simulink model "Figure_1_5_TP_Telecom_demodulation"  (R2020a)
settings: Solver=FixedStepDiscrete  StartTime=0.0  StopTime=999  RelTol=1e-3
libraries: simulink x2, commrandsrc3 x1, commsink2 x1, commfilt2 x1, dspsigops x1, commutil2 x1
Description:
  | C'est un TP Télécom à faire.
settings Model: Creator=Mr Ibrahima BA  LastModifiedBy=iba

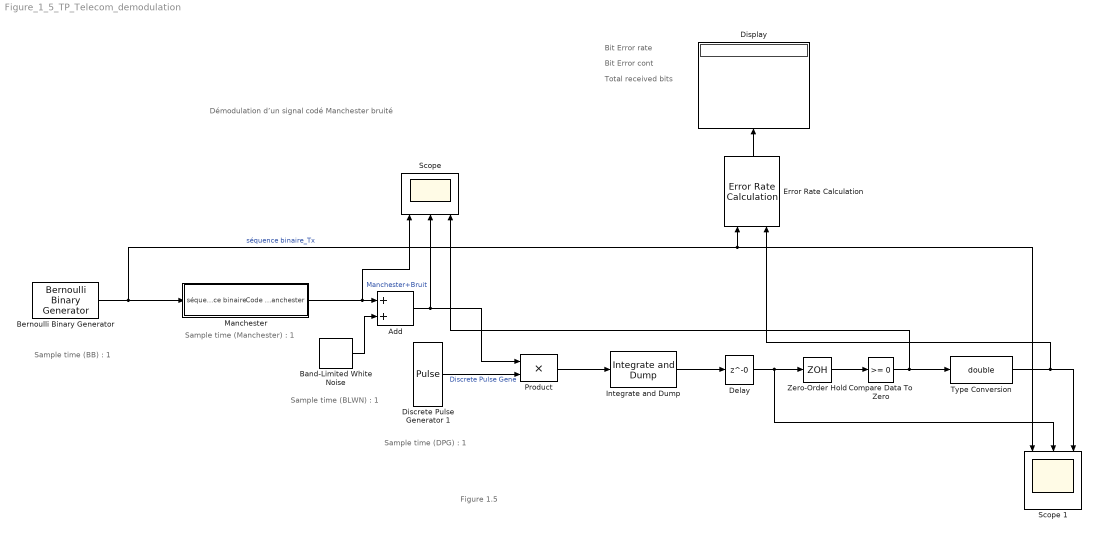
== system Figure_1_5_TP_Telecom_demodulation ==
  note: Sample time (BB) : 1
  note: Figure 1.5
  note: Démodulation d’un signal codé Manchester bruité
  note: Bit Error rate
  note: Bit Error cont
  note: Total received bits
  note: Sample time (Manchester) : 1
  note: Sample time (DPG) : 1
  note: Sample time (BLWN) : 1
  Add : Sum
  Band-Limited White Noise : simulink/Sources/Band-Limited White Noise  Cov=[1e-3]  Ts=0.1  seed=[23341]
  "Bernoulli Binary Generator " : commrandsrc3/Bernoulli Binary Generator  ProbabilityOfZero=0.5  SeedSource=Parameter  Seed=25.  SampleTime=1  SamplesPerFrame=1  OutputDataType=double  SimulateUsing=Interpreted execution
  Compare Data To Zero : simulink/Logic and Bit Operations/Compare To Zero  relop=>=  OutDataTypeStr=uint8  ZeroCross=off
  Delay : Delay  DelayLength=0
  "Discrete Pulse Generator 1 " : DiscretePulseGenerator  Period=1  SampleTime=0.5
  Display : Display
  "Error Rate Calculation " : commsink2/Error Rate Calculation  N=0  st_delay=0  cp_mode=Entire frame  subframe=[]  PMode=Port  WsName=ErrorVec  RsMode2=off  stop=off  numErr=100  maxBits=1000
  "Integrate and Dump " : commfilt2/Integrate and Dump  obssamples=10  offsetsamples=0  nodump=on  roundingMode=Floor  overflowMode=off  outputDataTypeStr=Inherit: Same as accumulator  outputLastDataTypeStr=Inherit: Same as accumulator
  Manchester : Subsystem
  "Product " : Product
  Scope : Scope  NumInputPorts=3
  Scope 1 : Scope  NumInputPorts=3
  Type Conversion : DataTypeConversion  OutDataTypeStr=double
  Zero-Order Hold : ZeroOrderHold
  wires:
  "Bernoulli Binary Generator "/1 -> Scope 1/1, "Error Rate Calculation "/1, Manchester/1(séquence binaire)  "séquence binaire_Tx"
  Band-Limited White Noise/1 -> Add/2
  "Discrete Pulse Generator 1 "/1 -> "Product "/2  "Discrete Pulse Gene"
  Add/1 -> "Product "/1, Scope/2  "Manchester+Bruit"
  "Product "/1 -> "Integrate and Dump "/1
  "Integrate and Dump "/1 -> Delay/1
  Compare Data To Zero/1 -> Scope/3, Type Conversion/1
  Type Conversion/1 -> Scope 1/3, "Error Rate Calculation "/2
  Manchester/1(Code Manchester) -> Scope/1, Add/1
  "Error Rate Calculation "/1 -> Display/1
  Zero-Order Hold/1 -> Compare Data To Zero/1
  Delay/1 -> Scope 1/2, Zero-Order Hold/1

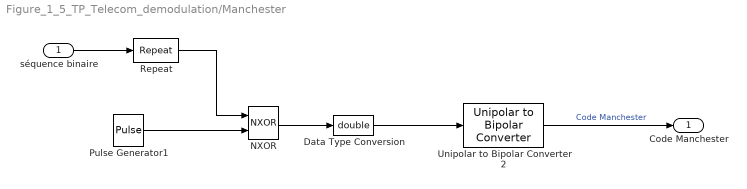
== system Figure_1_5_TP_Telecom_demodulation/Manchester ==
  séquence binaire : Inport
  "Data Type Conversion " : DataTypeConversion  OutDataTypeStr=double  LockScale=on
  NXOR : Logic  Operator=NXOR  AllPortsSameDT=off  OutDataTypeStr=boolean
  Pulse Generator1 : DiscretePulseGenerator  SampleTime=0.5
  Repeat : dspsigops/Repeat  N=2  RateOptions=Allow multirate processing  ic=0  mode=Unused parameter value
  Unipolar to Bipolar Converter 2 : commutil2/Unipolar to Bipolar Converter  M=2  polarity=Positive  dataType=Inherit via internal rule
  Code Manchester : Outport
  wires:
  Pulse Generator1/1 -> NXOR/2
  NXOR/1 -> "Data Type Conversion "/1
  séquence binaire/1 -> Repeat/1
  "Data Type Conversion "/1 -> Unipolar to Bipolar Converter 2/1
  Unipolar to Bipolar Converter 2/1 -> Code Manchester/1  "Code Manchester"
  Repeat/1 -> NXOR/1
